simulink model "VHF_central_unit"  (R2024a)
settings: Solver=FixedStepDiscrete  StartTime=0.0  StopTime=10.0  FixedStep=0.001  RelTol=1e-3  EnableMultiTasking=on
PreLoadFcn:
  | try
  | MDL_install;
  | catch
  | end
InitFcn:
  | EcoCoder_PreCheckLic();
undefined symbols (not defined in the file or in its folder): C_ROTSPD_ZERO, C_SOC_ZERO, h, km, s, V
libraries: CoderSF_BSW_Libs x222, SF_CanService_Libs x16, CoderSF_ADC2Volt_Libs x6, CoderSF_6AxisMEMS_Libs x6, canmsglib x3, EV_ASWLibs x2, simulink x2, Chassis_stability_controllers x1, CoderSF_KeyCycle_Libs x1
(part 4 of 4)

== system VHF_central_unit/ASW_Demo/01  process input signals/02 process driver input signals/02 process driver input signals/03 processs accelerator pedal/02 voltage selection/SelSig_GetStSigSrc ==
  diagDrvPedacc1_flgShrtPwr : Inport
  diagDrvPedacc2_flgShrtPwr : Inport  Port=2
  diagDrvPedacc1_flgFinalDef : Inport  Port=3
  diagDrvPedacc2_flgFinalDef : Inport  Port=4
  diagDrvPedacc_flgSyncDef : Inport  Port=5
  Constant : Constant  Value=0  OutDataTypeStr=Inherit: Inherit via back propagation  SampleTime=-1
  Terminator{,1..4} (5 alike) : Terminator
  sigInDrvPedacc_stSigSrc : Outport
  wires:
  diagDrvPedacc_flgSyncDef/1 -> Terminator4/1
  diagDrvPedacc2_flgFinalDef/1 -> Terminator3/1
  diagDrvPedacc1_flgFinalDef/1 -> Terminator2/1
  diagDrvPedacc2_flgShrtPwr/1 -> Terminator1/1
  diagDrvPedacc1_flgShrtPwr/1 -> Terminator/1
  Constant/1 -> sigInDrvPedacc_stSigSrc/1  "sigInDrvPedacc_stSigSrc"

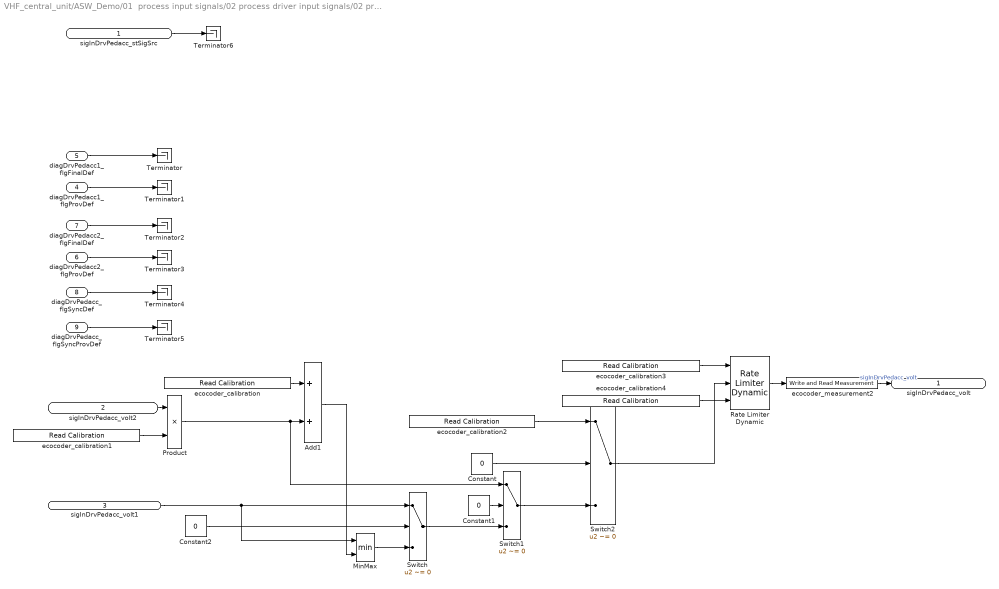
== system VHF_central_unit/ASW_Demo/01  process input signals/02 process driver input signals/02 process driver input signals/03 processs accelerator pedal/02 voltage selection/SelSig_GetURaw ==
  sigInDrvPedacc_stSigSrc : Inport
  sigInDrvPedacc_volt2 : Inport  Port=2
  sigInDrvPedacc_volt1 : Inport  Port=3
  diagDrvPedacc1_flgProvDef : Inport  Port=4
  diagDrvPedacc1_flgFinalDef : Inport  Port=5
  diagDrvPedacc2_flgProvDef : Inport  Port=6
  diagDrvPedacc2_flgFinalDef : Inport  Port=7
  diagDrvPedacc_flgSyncDef : Inport  Port=8
  diagDrvPedacc_flgSyncProvDef : Inport  Port=9
  Add1 : Sum  RndMeth=Simplest  SaturateOnIntegerOverflow=on  OutDataTypeStr=Inherit: Same as first input
  Constant : Constant  Value=0  OutDataTypeStr=Inherit: Inherit via back propagation  SampleTime=-1
  Constant1 : Constant  Value=0  OutDataTypeStr=Inherit: Inherit via back propagation  SampleTime=-1
  Constant2 : Constant  Value=0  OutDataTypeStr=Inherit: Inherit via back propagation  SampleTime=-1
  MinMax : MinMax  Inputs=2
  Product : Product  OutDataTypeStr=Inherit: Inherit via back propagation  RndMeth=Simplest  SaturateOnIntegerOverflow=on
  Rate Limiter Dynamic : simulink/Discontinuities/Rate Limiter Dynamic
  Switch : Switch  Criteria=u2 ~= 0  RndMeth=Simplest  InputSameDT=off
  Switch1 : Switch  Criteria=u2 ~= 0  RndMeth=Simplest  InputSameDT=off
  Switch2 : Switch  Criteria=u2 ~= 0  RndMeth=Simplest  InputSameDT=off
  Terminator{,1..6} (7 alike) : Terminator
  ecocoder_calibration : CoderSF_BSW_Libs/Calibration & Measurement/Read Calibration  variable_name=sigInDrvPedacc2_voltOffset_val  variable_value=0  variable_type=single  variable_min=[]  variable_max=[]  unitStr=V  descStr=""
      settings: AttributesFormatString=value:%<variable_value> type:%<variable_type> max:%<variable_max> Min:%<variable_min>
  ecocoder_calibration1 : CoderSF_BSW_Libs/Calibration & Measurement/Read Calibration  variable_name=sigInDrvPedacc_dRawSigFac_val  variable_value=0  variable_type=single  variable_min=[]  variable_max=[]  unitStr=""  descStr=""
      settings: AttributesFormatString=value:%<variable_value> type:%<variable_type> max:%<variable_max> Min:%<variable_min>
  ecocoder_calibration2 : CoderSF_BSW_Libs/Calibration & Measurement/Read Calibration  variable_name=sigInDrvPedacc_voltDef_val  variable_value=0  variable_type=single  variable_min=[]  variable_max=[]  unitStr=V  descStr=""
      settings: AttributesFormatString=value:%<variable_value> type:%<variable_type> max:%<variable_max> Min:%<variable_min>
  ecocoder_calibration3 : CoderSF_BSW_Libs/Calibration & Measurement/Read Calibration  variable_name=sigInDrvPedacc_dvoltLimErrPos_val  variable_value=0  variable_type=single  variable_min=[]  variable_max=[]  unitStr=V/s  descStr=""
      settings: AttributesFormatString=value:%<variable_value> type:%<variable_type> max:%<variable_max> Min:%<variable_min>
  ecocoder_calibration4 : CoderSF_BSW_Libs/Calibration & Measurement/Read Calibration  variable_name=sigInDrvPedacc_dvoltLimErrNeg_val  variable_value=0  variable_type=single  variable_min=[]  variable_max=[]  unitStr=V/s  descStr=""
      settings: AttributesFormatString=value:%<variable_value> type:%<variable_type> max:%<variable_max> Min:%<variable_min>
  ecocoder_measurement2 : CoderSF_BSW_Libs/Calibration & Measurement/Write and Read Measurement  variable_name=sigInDrvPedacc_volt  variable_value=0  variable_type=single  numD=1  unitStr=V  descStr=""
      settings: AttributesFormatString=value:%<variable_value> type:%<variable_type>
  sigInDrvPedacc_volt : Outport
  wires:
  sigInDrvPedacc_stSigSrc/1 -> Terminator6/1
  diagDrvPedacc1_flgFinalDef/1 -> Terminator/1
  diagDrvPedacc1_flgProvDef/1 -> Terminator1/1
  diagDrvPedacc2_flgFinalDef/1 -> Terminator2/1
  diagDrvPedacc2_flgProvDef/1 -> Terminator3/1
  diagDrvPedacc_flgSyncProvDef/1 -> Terminator5/1
  diagDrvPedacc_flgSyncDef/1 -> Terminator4/1
  sigInDrvPedacc_volt2/1 -> Product/1
  ecocoder_calibration/1 -> Add1/1
  ecocoder_calibration1/1 -> Product/2
  sigInDrvPedacc_volt1/1 -> Switch/1, MinMax/1
  MinMax/1 -> Switch/3
  Add1/1 -> MinMax/2
  ecocoder_calibration2/1 -> Switch2/1
  Switch/1 -> Switch1/3
  Constant2/1 -> Switch/2
  Constant1/1 -> Switch1/2
  Constant/1 -> Switch2/2
  ecocoder_calibration3/1 -> Rate Limiter Dynamic/1
  Switch1/1 -> Switch2/3
  Switch2/1 -> Rate Limiter Dynamic/2
  Rate Limiter Dynamic/1 -> ecocoder_measurement2/1
  ecocoder_calibration4/1 -> Rate Limiter Dynamic/3
  Product/1 -> Add1/2, Switch1/1
  ecocoder_measurement2/1 -> sigInDrvPedacc_volt/1  "sigInDrvPedacc_volt"

== system VHF_central_unit/ASW_Demo/01  process input signals/02 process driver input signals/02 process driver input signals/03 processs accelerator pedal/03 convert voltage to percentage/GetRUnFlt ==
  sigInDrvPedacc_volt : Inport
  Delay : Delay  DelayLength=1
  GetRUnFlt_Unjitter : Subsystem  TreatAsAtomicUnit=on
      settings: RTWSystemCode=Nonreusable function  RTWFcnNameOpts=Use subsystem name
  Subtract : Sum  Inputs=+-  RndMeth=Simplest  SaturateOnIntegerOverflow=on
  ecocoder_calibration : CoderSF_BSW_Libs/Calibration & Measurement/Read Calibration  variable_name=sigInDrvPedacc_voltJitter_val  variable_value=0  variable_type=single  variable_min=[]  variable_max=[]  unitStr=V  descStr=""
      settings: AttributesFormatString=value:%<variable_value> type:%<variable_type> max:%<variable_max> Min:%<variable_min>
  ecocoder_calibration1 : CoderSF_BSW_Libs/Calibration & Measurement/Read Calibration  variable_name=sigInDrvPedacc_flgtEnaUnJit_val  variable_value=0  variable_type=single  variable_min=[]  variable_max=[]  unitStr=""  descStr=""
      settings: AttributesFormatString=value:%<variable_value> type:%<variable_type> max:%<variable_max> Min:%<variable_min>
  ecocoder_measurement : CoderSF_BSW_Libs/Calibration & Measurement/Write and Read Measurement  variable_name=sigInDrvPedacc_pctUnFlt  variable_value=0  variable_type=single  numD=1  unitStr=""  descStr=""
      settings: AttributesFormatString=value:%<variable_value> type:%<variable_type>
  ecocoder_measurement1 : CoderSF_BSW_Libs/Calibration & Measurement/Write and Read Measurement  variable_name=sigInDrvPedacc_dpctUnFlt  variable_value=0  variable_type=single  numD=1  unitStr=V/20ms  descStr=""
      settings: AttributesFormatString=value:%<variable_value> type:%<variable_type>
  "sigInDrvPedacc_pctLin_cur " : CoderSF_BSW_Libs/Calibration & Measurement/1-D Lookup Table  nam=sigInDrvPedacc_pctLin  breakpoint_type=single  breakpoint_data=[0.3000 4.8000]  table_type=single  table_data=[0 1]
  sigInDrvPedacc_dpctUnFlt : Outport
  sigInDrvPedacc_pctUnFlt : Outport  Port=2
  wires:
  "sigInDrvPedacc_pctLin_cur "/1 -> ecocoder_measurement/1, Subtract/1, Delay/1
  Subtract/1 -> ecocoder_measurement1/1
  Delay/1 -> Subtract/2
  sigInDrvPedacc_volt/1 -> GetRUnFlt_Unjitter/1(sigInDrvPedacc_volt)
  ecocoder_calibration/1 -> GetRUnFlt_Unjitter/2(sigInDrvPedacc_voltJitter_val)
  GetRUnFlt_Unjitter/1(sigInDrvPedacc_voltUnJit) -> "sigInDrvPedacc_pctLin_cur "/1
  ecocoder_calibration1/1 -> GetRUnFlt_Unjitter/3(sigInDrvPedacc_flgtEnaUnJit_val)
  ecocoder_measurement/1 -> sigInDrvPedacc_pctUnFlt/1  "sigInDrvPedacc_pctUnFlt"
  ecocoder_measurement1/1 -> sigInDrvPedacc_dpctUnFlt/1  "sigInDrvPedacc_dpctUnFlt"

== system VHF_central_unit/ASW_Demo/01  process input signals/02 process driver input signals/02 process driver input signals/03 processs accelerator pedal/03 convert voltage to percentage/GetRUnFlt/GetRUnFlt_Unjitter ==
  sigInDrvPedacc_volt : Inport
  sigInDrvPedacc_voltJitter_val : Inport  Port=2
  sigInDrvPedacc_flgtEnaUnJit_val : Inport  Port=3
  DT_conv1 : DataTypeConversion  SaturateOnIntegerOverflow=off  RndMeth=Floor
  Terminator : Terminator
  Terminator1 : Terminator
  ecocoder_measurement : CoderSF_BSW_Libs/Calibration & Measurement/Write and Read Measurement  variable_name=sigInDrvPedacc_voltUnJit  variable_value=0  variable_type=single  numD=1  unitStr=V  descStr=""
      settings: AttributesFormatString=value:%<variable_value> type:%<variable_type>
  sigInDrvPedacc_voltUnJit : Outport
  wires:
  DT_conv1/1 -> ecocoder_measurement/1
  sigInDrvPedacc_voltJitter_val/1 -> Terminator/1
  sigInDrvPedacc_flgtEnaUnJit_val/1 -> Terminator1/1
  sigInDrvPedacc_volt/1 -> DT_conv1/1
  ecocoder_measurement/1 -> sigInDrvPedacc_voltUnJit/1  "sigInDrvPedacc_voltUnJit"
